simulink model "ds_simple_twozone"  (R2020a)
settings: Solver=ode1be  StartTime=0.0  StopTime=Inf  FixedStep=0.001  RelTol=1e-3
PostLoadFcn:
  | if any(exist('dsrtsu_mdlpostloadfcn', 'file') ~= 0), dsrtsu_mdlpostloadfcn('Execute', bdroot); end
InitFcn:
  | , if any(exist('rtifpga_mdlclblib', 'file') ~= 0), rtifpga_mdlclblib('Init', bdroot); end,
  | , if any(exist('dsmpb_private', 'file') ~= 0), dsmpb_private('dsmpb_mdlclblib', 'Init', bdroot); end,
libraries: neural x7, dsmpblib x7
(part 1 of 3)
PreSaveFcn:
  | , if any(exist('dsmpb_private', 'file') ~= 0), dsmpb_private('dsmpb_mdlclblib', 'PreSave', bdroot); end,
CloseFcn:
  | , if any(exist('dsmpb_private', 'file') ~= 0), dsmpb_private('dsmpb_mdlclblib', 'Close', bdroot); end,
settings Model: RTICANMMDATA=struct('GeneralSetupData',struct('modelroot','D:\github\dspace-modelica-example\dSpaceExample','generalsettings',struct('filesettings',struct('destfolder',struct('Name','RTICANMM_FILES','Check',1),'buildfolder',struct('Name','.','Check',1),'AbsDestfolder',struct('Name','D:\github\dspace-modelica-example\dSpaceExample\RTICANMM_FILES'),'AbsBuildfolder',struct('Name','D:\github\dspace-modelica-example\dSpaceExample'))),'options',struct('addpaths',1,'rmpaths',1,'addtrcexclusion',true,'cannavigator',struct('checkmonitoring',0),'show_usrtrc',0,'use_usrtrc',0),'advanced',struct('options',ones(1,100)),'MPSetup',{{}},'RTI',struct('Type','DSRT','Ver','4.3','Date','02-May-2020'),'modelname','ds_simple_twozone','block','ds_simple_twozone'))  DSRTSU_INTERNAL_RTIFPGA=160  DSMPB_ID_DATA={'132',struct('BlockId','fbc3f0c5-b68b-4d01-9f2d-36209dda977c','SignalIds',{{'ca641e27-4795-4c1e-9df1-2cbc48e7930b'}}),'133',struct('BlockId','70872080-617a-4356-af6c-b8420dd1a1f8','SignalIds',{{'3418c3fd-757d-4941-a689-5502bdc455a5'}}),'134',struct('BlockId','85d3d815-1754-4189-8dca-79ff9754a612','SignalIds',{{'e8f6075e-0c9a-4051-a7fe-ef09ffc889a6'}}),'135',struct('BlockId','5ea4ccaf-109d-448b-a418-88c7068c4cdc','SignalIds',{{'cf95ed01-646a-4606-82e3-1eeb14ab658a'}}),'136',struct('BlockId','d022eeec-8516-4a23-9d10-dc3252dc1678','SignalIds',{{'ed65049e-3e32-4616-921d-83e7805a173d'}}),'137',struct('BlockId','a079a78e-6021-4250-821f-e2536e68fe73','SignalIds',{{'c9129c4d-d3a0-4e83-aef0-658117b44ff4'}}),'138',struct('BlockId','7105b817-1da7-4089-b5b1-06748f49c5e5','SignalIds',{{'d0544b60-35f0-4f17-87a7-41ea08d9345b'}}),'139',struct('BlockId','3e88e1ee-0445-4382-b044-7e2487c4b054','SignalIds',{{'65da7ff3-6d35-41d2-be02-8ae6c002fa6b'}}),'236',struct('BlockId','db60070b-df7b-44ed-b750-cfd2b2fb3f9f','SignalIds',{{'bb3a5f76-9421-4e74-869d-1121775f016d'}}),'237',struct('BlockId','e9b9945a-31f3-4010-a8f7-35b42b310d19','SignalIds',{{'9f4600a4-f050-4de3-b65c-a4e916c07273'}}),'238',struct('BlockId','2c11abef-c5d0-4944-bc68-9310ebf6e01f','SignalIds',{{'04ba7a63-2602-44d5-947f-4ac2f5006d2b'}}),'239',struct('BlockId','d057b1e2-fe3b-4b69-9a22-ac3e68195dda','SignalIds',{{'77330597-c16e-4df2-9510-155471efb7bd'}}),'240',struct('BlockId','08f95fd0-40cf-47d5-ab4c-59a75cfa282c','SignalIds',{{'eadba8ad-2dab-4e97-8c0a-c4e323ad4b42'}}),'241',struct('BlockId','b5e1c2c7-b317-4633-bd12-793f49455b19','SignalIds',{{'9e9eef31-2180-474d-8328-a0ce75ef502c'}}),'242',struct('BlockId','be52a969-daf4-4d41-81e7-d2965b038824','SignalIds',{{'88cc5638-5a4d-4050-80e5-e1a520294fcc'}})}  Creator=yangyang.fu  LastModifiedBy=yangyang.fu
settings OptimizationCC: BlockReduction=off  ConditionallyExecuteInputs=off  OptimizeBlockIOStorage=off  BufferReuse=off
settings DebuggingCC: TasksWithSamePriorityMsg=none
settings HardwareCC: ProdBitPerPointer=32  ProdBitPerSizeT=32  ProdBitPerPtrDiffT=32  ProdLargestAtomicInteger=Integer  ProdWordSize=32  ProdLongLongMode=on  ProdHWDeviceType=Custom Processor->Custom
settings ModelReferenceCC: EnableParallelModelReferenceBuilds=on
settings SFSimCC: MATLABDynamicMemAlloc=off
settings RTWCC: Description=dSPACE Run-Time Target (for VEOS on Windows and ConfigurationDesk)  SystemTargetFile=dsrt.tlc  GenCodeOnly=on  MakeCommand=make_dsrt  TemplateMakefile=dsrt_default_tmf  RTWVerbose=off  CustomInclude="\"C:\\Program Files\\Dymola 2021\\Source\""
settings STFCustomTargetCC: TargetLangStandard=C99 (ISO)  ParMdlRefBuildCompliant=on  SystemTargetFile=dsrt.tlc
settings GRTTargetCC: CompOptLevelCompliant=off  ConcurrentExecutionCompliant=off  CombineOutputUpdateFcns=off  MatFileLogging=off  CPPClassGenCompliant=off  UseToolchainInfoCompliant=off

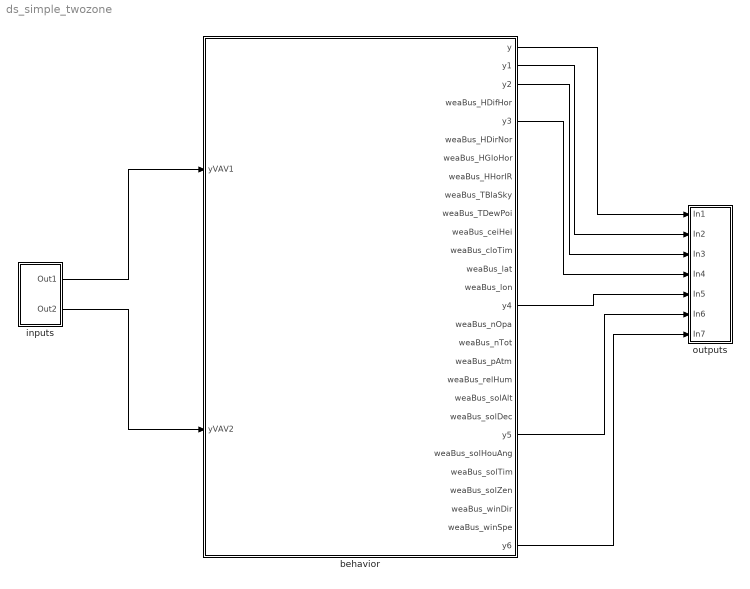
== system ds_simple_twozone ==
  behavior : Subsystem
  inputs : Subsystem
  outputs : Subsystem
  wires:
  inputs/1(Out1) -> behavior/1(yVAV1)
  inputs/2(Out2) -> behavior/2(yVAV2)
  behavior/1(y) -> outputs/1(In1)
  behavior/2(y1) -> outputs/2(In2)
  behavior/3(y2) -> outputs/3(In3)
  behavior/5(y3) -> outputs/4(In4)
  behavior/15(y4) -> outputs/5(In5)
  behavior/22(y5) -> outputs/6(In6)
  behavior/28(y6) -> outputs/7(In7)

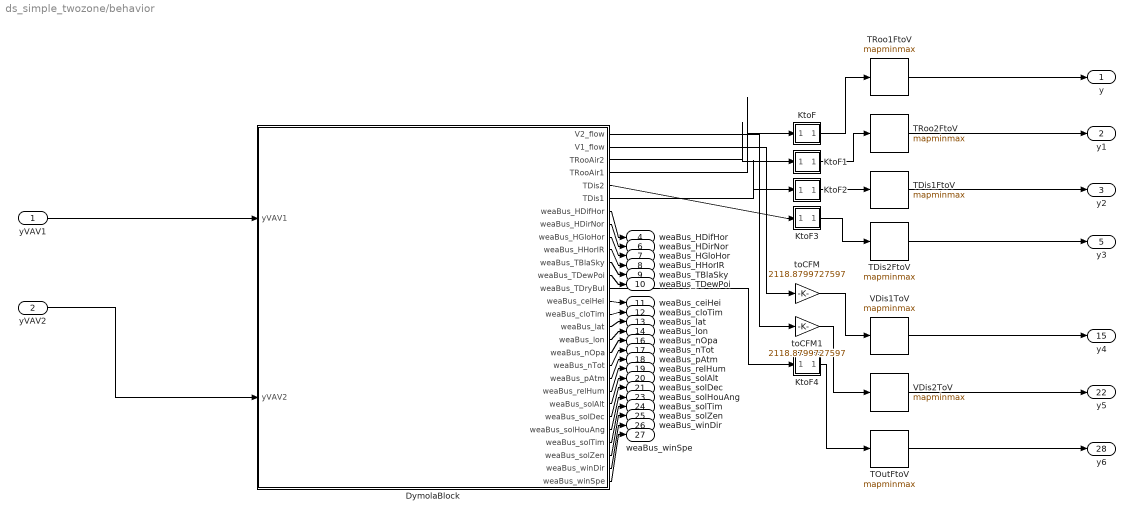
== system ds_simple_twozone/behavior ==
  yVAV1 : Inport
  yVAV2 : Inport  Port=2
  DymolaBlock : Subsystem  Tag=11-Oct-2021 17:25:52#4854
      mask help:
      | Dymola block.
      | A dymola block allows acausal physical modeling.
      | See Dymola manual for usage.
      settings: CopyFcn=newDymolaGui('11-Oct-2021 17:25:52#4854','Copy');  DeleteFcn=if exist('newDymolaGui') newDymolaGui('ds_simple_twozone/behavior/DymolaBlock','Delete'); end;  NameChangeFcn=newDymolaGui('11-Oct-2021 17:25:52#4854','Copy');  OpenFcn=newDymolaGui('ds_simple_twozone/behavior/DymolaBlock','Init');
      mask Display: image(reshape([1;1;1;1;1;1;1;1;1;1;1;1;1;1;1;1;1;1;1;1;1;1;0;0;0;0;0;0;0;0;0;0;1;1;1;1;1;1;1;1;0;1;1;1;1;1;1;1;1;0;1;1;1;1;1;0;0;0;0;0;0;0;1;1;0;0;0;0;0;0;0;1;1;0;0;0;0;0;0;0;1;1;0;0;0;0;0;0;0;1;1;0;0;0;0;0;0;0;1;1;0;0;0;0;0;0;0;1;1;0;0;0;0;0;0;0;1;1;0;0;0;0;0;0;0;1;1;0;0;0;0;0;0;0;1;1;0;0;0;0;0;0;0;1;1;0;0;0;0;0;0;0;1;1;0;0;0;0;0;0;0;1;1;0;0;0;0;0;0;0;1;1;0;0;0;0;0;0;0;1;1;0;0;0;0;0;0;0;1;1;0;0;0;0;0;0;0;1;1;0;0;0;0;0;0;0;1;1;0;0;0;0;0;0;0;1;1;0;0;0;0;0;0;0;1;1;0;0;0;0;0;0;0;1;1;0;0;0;0;0;0;0;1;1;0;0;0;0;0;0;0;1;1;0;0;0;0;0;0;0;1;1;0;0;0;0;0;0;0;1;1;1;1;1;0;1;1;1;1;1;1;1;1;0;1;1;1;1;1;1;1;1;0;0;0;0;0;0;0;0;0;0;1;1;1;1;1;1;1;1;1;1;1;1;1;1;1;1;1;1;1;1;1;1;1;1;1;1;1;1;1;1;1;1;1;1;1;1;1;1;1;1;1;1;1;1;0;0;0;0;0;0;0;0;0;0;1;1;1;1;1;1;1;1;0;1;1;1;1;1;1;1;1;0;1;1;1;1;1;0;0;0;0;0;0;0;1;1;0;0;0;0;0;0;0;1;1;0;0;0;0;0;0;0;1;1;0;0;0;0;0;0;0;1;1;0;0;0;0;0;0;0;1;1;0;0;0;0;0;0;0;1;1;0;0;0;0;0;0;0;1;1;0;0;0;0;0;0;0;1;1;0;0;0;0;0;0;0;1;1;0;0;0;0;0;0;0;1;1;0;0;0;0;0;0;0;1;1;0;0;0;0;0;0;0;1;1;0;0;0;0;0;0;0;1;1;0;0;0;0;0;0;0;1;1;0;0;0;0;0;0;0;1;1;0;0;0;0;0;0;0;1;1;0;0;0;0;0;0;0;1;1;0;0;0;0;0;0;0;1;1;0;0;0;0;0;0;0;1;1;0;0;0;0;0;0;0;1;1;0;0;0;0;0;0;0;1;1;0;0;0;0;0;0;0;1;1;0;0;0;0;0;0;0;1;1;0;0;0;0;0;0;0;1;1;1;1;1;0;1;1;1;1;1;1;1;1;0;1;1;1;1;1;1;1;1;0;0;0;0;0;0;0;0;0;0;1;1;1;1;1;1;1;1;1;1;1;1;1;1;1;1;1;1;1;1;1;1;1;1;1;1;1;1;1;1;1;1;1;1;1;1;1;1;1;1;1;1;1;1;0;0;0;0;0;0;0;0;0;0;1;1;1;1;1;1;1;1;0;1;1;1;1;1;1;1;1;0;1;1;1;1;1;0;0;0;0;0;0;0;1;1;0;0;0;0;0;0;0;1;1;0;1;1;1;1;1;0;1;1;0;1;1;1;1;1;0;1;1;0;1;1;1;1;1;0;1;1;0;1;1;1;1;1;0;1;1;0;1;1;1;1;1;0;1;1;0;1;1;1;1;1;0;1;1;0;1;1;1;1;1;0;1;1;0;1;1;1;1;1;0;1;1;0;1;1;1;1;1;0;1;1;0;1;1;1;1;1;0;1;1;0;1;1;1;1;1;0;1;1;0;1;1;1;1;1;0;1;1;0;1;1;1;1;1;0;1;1;0;1;1;1;1;1;0;1;1;0;1;1;1;1;1;0;1;1;0;1;1;1;1;1;0;1;1;0;1;1;1;1;1;0;1;1;0;1;1;1;1;1;0;1;1;0;1;1;1;1;1;0;1;1;0;1;1;1;1;1;0;1;1;0;0;0;0;0;0;0;1;1;0;0;0;0;0;0;0;1;1;1;1;1;0;1;1;1;1;1;1;1;1;0;1;1;1;1;1;1;1;1;0;0;0;0;0;0;0;0;0;0;1;1;1;1;1;1;1;1;1;1;1;1;1;1;1;1;1;1;1;1;1;1],18,18,3),[.2,.2,.6,.6])
  KtoF : Subsystem
  KtoF1 : Subsystem
  KtoF2 : Subsystem
  KtoF3 : Subsystem
  KtoF4 : Subsystem
  TDis1FtoV : neural/Processing Functions/mapminmax  xmin=-150  xmax=150  ymin=-10  ymax=+10
  TDis2FtoV : neural/Processing Functions/mapminmax  xmin=-150  xmax=150  ymin=-10  ymax=+10
  TOutFtoV : neural/Processing Functions/mapminmax  xmin=-150  xmax=150  ymin=-10  ymax=+10
  TRoo1FtoV : neural/Processing Functions/mapminmax  xmin=-150  xmax=150  ymin=-10  ymax=+10
  TRoo2FtoV : neural/Processing Functions/mapminmax  xmin=-150  xmax=150  ymin=-10  ymax=+10
  VDis1ToV : neural/Processing Functions/mapminmax  xmin=0  xmax=20000  ymin=-10  ymax=+10
  VDis2ToV : neural/Processing Functions/mapminmax  xmin=0  xmax=20000  ymin=-10  ymax=+10
  toCFM : Gain  Gain=2118.8799727597
  toCFM1 : Gain  Gain=2118.8799727597
  y : Outport
  y1 : Outport  Port=2
  y2 : Outport  Port=3
  weaBus_HDifHor : Outport  Port=4
  y3 : Outport  Port=5
  weaBus_HDirNor : Outport  Port=6
  weaBus_HGloHor : Outport  Port=7
  weaBus_HHorIR : Outport  Port=8
  weaBus_TBlaSky : Outport  Port=9
  weaBus_TDewPoi : Outport  Port=10
  weaBus_ceiHei : Outport  Port=11
  weaBus_cloTim : Outport  Port=12
  weaBus_lat : Outport  Port=13
  weaBus_lon : Outport  Port=14
  y4 : Outport  Port=15
  weaBus_nOpa : Outport  Port=16
  weaBus_nTot : Outport  Port=17
  weaBus_pAtm : Outport  Port=18
  weaBus_relHum : Outport  Port=19
  weaBus_solAlt : Outport  Port=20
  weaBus_solDec : Outport  Port=21
  y5 : Outport  Port=22
  weaBus_solHouAng : Outport  Port=23
  weaBus_solTim : Outport  Port=24
  weaBus_solZen : Outport  Port=25
  weaBus_winDir : Outport  Port=26
  weaBus_winSpe : Outport  Port=27
  y6 : Outport  Port=28
  wires:
  KtoF3/1(Out1) -> TDis2FtoV/1
  DymolaBlock/11(weaBus_TBlaSky) -> weaBus_TBlaSky/1
  DymolaBlock/5(TDis2) -> KtoF3/1(In1)
  DymolaBlock/2(V1_flow) -> toCFM/1
  DymolaBlock/8(weaBus_HDirNor) -> weaBus_HDirNor/1
  DymolaBlock/24(weaBus_solHouAng) -> weaBus_solHouAng/1
  KtoF/1(Out1) -> TRoo1FtoV/1
  DymolaBlock/1(V2_flow) -> toCFM1/1
  KtoF4/1(Out1) -> TOutFtoV/1
  DymolaBlock/14(weaBus_ceiHei) -> weaBus_ceiHei/1
  toCFM1/1 -> VDis2ToV/1
  DymolaBlock/12(weaBus_TDewPoi) -> weaBus_TDewPoi/1
  KtoF2/1(Out1) -> TDis1FtoV/1
  yVAV2/1 -> DymolaBlock/2(yVAV2)
  DymolaBlock/4(TRooAir1) -> KtoF/1(In1)
  DymolaBlock/3(TRooAir2) -> KtoF1/1(In1)
  KtoF1/1(Out1) -> TRoo2FtoV/1
  toCFM/1 -> VDis1ToV/1
  DymolaBlock/13(weaBus_TDryBul) -> KtoF4/1(In1)
  DymolaBlock/6(TDis1) -> KtoF2/1(In1)
  DymolaBlock/10(weaBus_HHorIR) -> weaBus_HHorIR/1
  DymolaBlock/9(weaBus_HGloHor) -> weaBus_HGloHor/1
  DymolaBlock/7(weaBus_HDifHor) -> weaBus_HDifHor/1
  DymolaBlock/19(weaBus_nTot) -> weaBus_nTot/1
  TDis2FtoV/1 -> y3/1
  TRoo1FtoV/1 -> y/1
  DymolaBlock/17(weaBus_lon) -> weaBus_lon/1
  DymolaBlock/18(weaBus_nOpa) -> weaBus_nOpa/1
  DymolaBlock/26(weaBus_solZen) -> weaBus_solZen/1
  DymolaBlock/15(weaBus_cloTim) -> weaBus_cloTim/1
  yVAV1/1 -> DymolaBlock/1(yVAV1)
  TDis1FtoV/1 -> y2/1
  TOutFtoV/1 -> y6/1
  DymolaBlock/23(weaBus_solDec) -> weaBus_solDec/1
  DymolaBlock/16(weaBus_lat) -> weaBus_lat/1
  VDis1ToV/1 -> y4/1
  DymolaBlock/21(weaBus_relHum) -> weaBus_relHum/1
  DymolaBlock/27(weaBus_winDir) -> weaBus_winDir/1
  DymolaBlock/20(weaBus_pAtm) -> weaBus_pAtm/1
  DymolaBlock/22(weaBus_solAlt) -> weaBus_solAlt/1
  DymolaBlock/25(weaBus_solTim) -> weaBus_solTim/1
  DymolaBlock/28(weaBus_winSpe) -> weaBus_winSpe/1
  VDis2ToV/1 -> y5/1
  TRoo2FtoV/1 -> y1/1

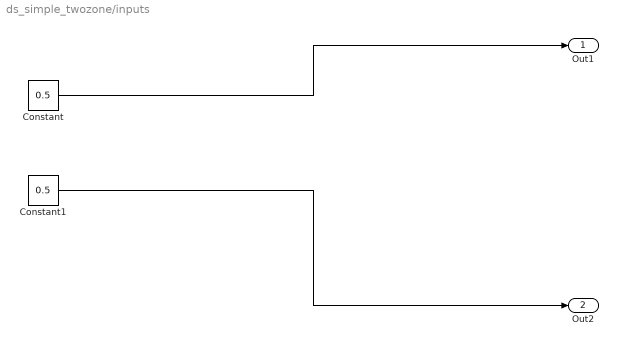
== system ds_simple_twozone/inputs ==
  Constant : Constant  Value=0.5  SampleTime=0.01
  Constant1 : Constant  Value=0.5  SampleTime=0.01
  Out1 : Outport
  Out2 : Outport  Port=2
  wires:
  Constant/1 -> Out1/1
  Constant1/1 -> Out2/1

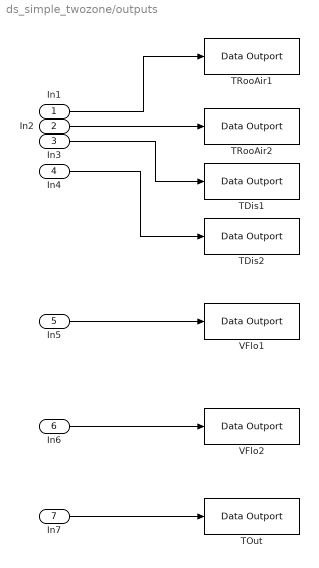
== system ds_simple_twozone/outputs ==
  In1 : Inport
  In2 : Inport  Port=2
  In3 : Inport  Port=3
  In4 : Inport  Port=4
  In5 : Inport  Port=5
  In6 : Inport  Port=6
  In7 : Inport  Port=7
  TDis1 : dsmpblib/Data Outport  Priority=-10000
      settings: SourceProductName=dSPACE Model Interface Blockset
  TDis2 : dsmpblib/Data Outport  Priority=-10000
      settings: SourceProductName=dSPACE Model Interface Blockset
  TOut : dsmpblib/Data Outport  Priority=-10000
      settings: SourceProductName=dSPACE Model Interface Blockset
  TRooAir1 : dsmpblib/Data Outport  Priority=-10000
      settings: SourceProductName=dSPACE Model Interface Blockset
  TRooAir2 : dsmpblib/Data Outport  Priority=-10000
      settings: SourceProductName=dSPACE Model Interface Blockset
  VFlo1 : dsmpblib/Data Outport  Priority=-10000
      settings: SourceProductName=dSPACE Model Interface Blockset
  VFlo2 : dsmpblib/Data Outport  Priority=-10000
      settings: SourceProductName=dSPACE Model Interface Blockset
  wires:
  In1/1 -> TRooAir1/1
  In2/1 -> TRooAir2/1
  In3/1 -> TDis1/1
  In4/1 -> TDis2/1
  In5/1 -> VFlo1/1
  In6/1 -> VFlo2/1
  In7/1 -> TOut/1
